simulink model "Final_Tune_of_Bandwidth_PI_Result"  (R2022b)
settings: Solver=FixedStepDiscrete  StartTime=0.0  StopTime=Inf  FixedStep=100e-6  RelTol=1e-3  EnableMultiTasking=on
undefined symbols (not defined in the file): C28x, CPU1, CPU2, CurrentBypassValue, DiscIntNeverNeededParam, Down, GPTRIP1SEL, TZ1, Up
libraries: c2802xlib x20, simulink x16, dspstat3 x10, dspsigops x6, c2837xDlib x5, PID_Lib x5, c280xlib x3, c2000lib x1
(part 3 of 3)

== system Final_Tune_of_Bandwidth_PI_Result/Subsystem5/Subsystem3 ==
  DiffInput : Inport
  Trigger : Inport  Port=2
  Cast1 : DataTypeConversion  OutDataTypeStr=int8  SaturateOnIntegerOverflow=off  RndMeth=Floor
  Mean1 : dspstat3/Mean  run=on  InputProcessing=Columns as channels (frame based)  reset_popup=Rising edge  directionMode=Each column  dimension=1  roiEnable=off  roiType=Rectangles  roiPortion=Entire ROI  roiOutput=Individual statistics for each ROI  roiFlag=off  roundingMode=Floor  overflowMode=off  outputDataTypeStr=Inherit: Same as accumulator  outputMin=[]  outputMax=[]  outputLastDataTypeStr=Inherit: Same as accumulator
  Mean : Outport
  wires:
  Cast1/1 -> Mean1/2
  DiffInput/1 -> Mean1/1
  Mean1/1 -> Mean/1
  Trigger/1 -> Cast1/1

== system Final_Tune_of_Bandwidth_PI_Result/Subsystem5/Subsystem4 ==
  DiffInput : Inport
  Trigger : Inport  Port=2
  Cast1 : DataTypeConversion  OutDataTypeStr=int8  SaturateOnIntegerOverflow=off  RndMeth=Floor
  Mean1 : dspstat3/Mean  run=on  InputProcessing=Columns as channels (frame based)  reset_popup=Rising edge  directionMode=Each column  dimension=1  roiEnable=off  roiType=Rectangles  roiPortion=Entire ROI  roiOutput=Individual statistics for each ROI  roiFlag=off  roundingMode=Floor  overflowMode=off  outputDataTypeStr=Inherit: Same as accumulator  outputMin=[]  outputMax=[]  outputLastDataTypeStr=Inherit: Same as accumulator
  Mean : Outport
  wires:
  Cast1/1 -> Mean1/2
  DiffInput/1 -> Mean1/1
  Mean1/1 -> Mean/1
  Trigger/1 -> Cast1/1

== system Final_Tune_of_Bandwidth_PI_Result/Subsystem5/Subsystem6 ==
  DiffInput : Inport
  Trigger : Inport  Port=2
  Cast1 : DataTypeConversion  OutDataTypeStr=int8  SaturateOnIntegerOverflow=off  RndMeth=Floor
  Mean1 : dspstat3/Mean  run=on  InputProcessing=Columns as channels (frame based)  reset_popup=Rising edge  directionMode=Each column  dimension=1  roiEnable=off  roiType=Rectangles  roiPortion=Entire ROI  roiOutput=Individual statistics for each ROI  roiFlag=off  roundingMode=Floor  overflowMode=off  outputDataTypeStr=Inherit: Same as accumulator  outputMin=[]  outputMax=[]  outputLastDataTypeStr=Inherit: Same as accumulator
  Mean : Outport
  wires:
  Cast1/1 -> Mean1/2
  DiffInput/1 -> Mean1/1
  Mean1/1 -> Mean/1
  Trigger/1 -> Cast1/1

== system Final_Tune_of_Bandwidth_PI_Result/Voltage_Loop/Subsystem5 ==
  MPCC_f32DCLink : Inport
  Cast To Single1 : DataTypeConversion  OutDataTypeStr=single  SaturateOnIntegerOverflow=off  RndMeth=Floor
  LPF : Subsystem
  MPCC_f32DCLinkFiltered : Outport
  wires:
  LPF/1(y_k) -> Cast To Single1/1
  MPCC_f32DCLink/1 -> LPF/1(u_k)
  Cast To Single1/1 -> MPCC_f32DCLinkFiltered/1  "Iau"

== system Final_Tune_of_Bandwidth_PI_Result/Subsystem1/ABCtoDQO/ABCtoDQOCurrent ==
  PI_f32GridCurrentA : Inport
  PI_f32GridCurrentB : Inport  Port=2
  PI_f32GridCurrentC : Inport  Port=3
  PI_f32ElectricalAngle : Inport  Port=4
  ABCtoO : Subsystem
  ABCtoQ : Subsystem
  ABCtoQ1 : Subsystem
  PI_f32DGridCurrent : Outport
  PI_f32QGridCurrent : Outport  Port=2
  PI_f32OGridCurrent : Outport  Port=3
  wires:
  ABCtoQ/1(PI_f32QGridCurrent) -> PI_f32QGridCurrent/1
  [PI_f32GridCurrentC] -> ABCtoQ/3(PI_f32GridCurrentC)
  PI_f32GridCurrentC/1 -> [PI_f32GridCurrentC]
  PI_f32GridCurrentA/1 -> [PI_f32GridCurrentA]
  [PI_f32GridCurrentB] -> ABCtoO/2(PI_f32GridCurrentB)
  [PI_f32GridCurrentA] -> ABCtoO/1(PI_f32GridCurrentA)
  [PI_f32ElectricalAngle] -> ABCtoQ/4(PI_f32ElectricalAngle)
  [PI_f32GridCurrentA] -> ABCtoQ/1(PI_f32GridCurrentA)
  [PI_f32GridCurrentC] -> ABCtoO/3(PI_f32GridCurrentC)
  [PI_f32GridCurrentB] -> ABCtoQ/2(PI_f32GridCurrentB)
  PI_f32ElectricalAngle/1 -> [PI_f32ElectricalAngle]
  PI_f32GridCurrentB/1 -> [PI_f32GridCurrentB]
  ABCtoQ1/1(MPCC_f32QGridVoltage) -> PI_f32DGridCurrent/1
  ABCtoO/1(PI_f32OGridCurrent) -> PI_f32OGridCurrent/1
  [PI_f32GridCurrentA] -> ABCtoQ1/1(MPCC_f32GridVoltageA)
  [PI_f32GridCurrentB] -> ABCtoQ1/2(MPCC_f32GridVoltageB)
  [PI_f32GridCurrentC] -> ABCtoQ1/3(MPCC_f32GridVoltageC)
  [PI_f32ElectricalAngle] -> ABCtoQ1/4(MPCC_f32ElectricalAngle)

== system Final_Tune_of_Bandwidth_PI_Result/Subsystem1/ABCtoDQO/ABCtoDQOVoltage ==
  PI_f32GridCurrentA : Inport
  PI_f32GridCurrentB : Inport  Port=2
  PI_f32GridCurrentC : Inport  Port=3
  PI_f32ElectricalAngle : Inport  Port=4
  ABCtoO : Subsystem
  ABCtoQ : Subsystem
  ABCtoQ1 : Subsystem
  PI_f32DGridCurrent : Outport
  PI_f32QGridCurrent : Outport  Port=2
  PI_f32OGridCurrent : Outport  Port=3
  wires:
  ABCtoQ/1(PI_f32QGridCurrent) -> PI_f32QGridCurrent/1
  [PI_f32GridCurrentC] -> ABCtoQ/3(PI_f32GridCurrentC)
  PI_f32GridCurrentC/1 -> [PI_f32GridCurrentC]
  PI_f32GridCurrentA/1 -> [PI_f32GridCurrentA]
  [PI_f32GridCurrentB] -> ABCtoO/2(PI_f32GridCurrentB)
  [PI_f32GridCurrentA] -> ABCtoO/1(PI_f32GridCurrentA)
  [PI_f32ElectricalAngle] -> ABCtoQ/4(PI_f32ElectricalAngle)
  [PI_f32GridCurrentA] -> ABCtoQ/1(PI_f32GridCurrentA)
  [PI_f32GridCurrentC] -> ABCtoO/3(PI_f32GridCurrentC)
  [PI_f32GridCurrentB] -> ABCtoQ/2(PI_f32GridCurrentB)
  PI_f32ElectricalAngle/1 -> [PI_f32ElectricalAngle]
  PI_f32GridCurrentB/1 -> [PI_f32GridCurrentB]
  ABCtoQ1/1(MPCC_f32QGridVoltage) -> PI_f32DGridCurrent/1
  ABCtoO/1(PI_f32OGridCurrent) -> PI_f32OGridCurrent/1
  [PI_f32GridCurrentA] -> ABCtoQ1/1(MPCC_f32GridVoltageA)
  [PI_f32GridCurrentB] -> ABCtoQ1/2(MPCC_f32GridVoltageB)
  [PI_f32GridCurrentC] -> ABCtoQ1/3(MPCC_f32GridVoltageC)
  [PI_f32ElectricalAngle] -> ABCtoQ1/4(MPCC_f32ElectricalAngle)

== system Final_Tune_of_Bandwidth_PI_Result/Subsystem1/ABCtoDQO/abc_dq ==
  theta : Inport
  a : Inport  Port=2
  b : Inport  Port=3
  c : Inport  Port=4
  Subsystem5 : Subsystem
  Subsystem6 : Subsystem
  Id : Outport
  Iq : Outport  Port=2
  wires:
  c/1 -> Subsystem5/3(In3)
  Subsystem5/2(Out2) -> Subsystem6/2(In2)
  b/1 -> Subsystem5/2(In2)
  theta/1 -> Subsystem6/3(theta)
  Subsystem6/1(Id) -> Id/1
  Subsystem5/1(Out1) -> Subsystem6/1(In1)
  Subsystem6/2(Iq) -> Iq/1
  a/1 -> Subsystem5/1(In1)

== system Final_Tune_of_Bandwidth_PI_Result/Subsystem1/ABCtoDQO/abc_dq1 ==
  theta : Inport
  a : Inport  Port=2
  b : Inport  Port=3
  c : Inport  Port=4
  Subsystem5 : Subsystem
  Subsystem6 : Subsystem
  Id : Outport
  Iq : Outport  Port=2
  wires:
  c/1 -> Subsystem5/3(In3)
  Subsystem5/2(Out2) -> Subsystem6/2(In2)
  b/1 -> Subsystem5/2(In2)
  theta/1 -> Subsystem6/3(theta)
  Subsystem6/1(Id) -> Id/1
  Subsystem5/1(Out1) -> Subsystem6/1(In1)
  Subsystem6/2(Iq) -> Iq/1
  a/1 -> Subsystem5/1(In1)

== system Final_Tune_of_Bandwidth_PI_Result/Subsystem1/Decoupling_Loop/ABCtoDQOVoltage ==
  PI_f32MDVoltageRef : Inport
  PI_f32MQVoltageRef : Inport  Port=2
  PI_f32MOVoltageRef : Inport  Port=3
  PI_f32ElectricalAngle : Inport  Port=4
  DQOtoA : Subsystem
  DQOtoB : Subsystem
  DQOtoC : Subsystem
  PI_f32MAVoltageRef : Outport
  PI_f32MBVoltageRef : Outport  Port=2
  PI_f32MCVoltageRef : Outport  Port=3
  wires:
  [PI_f32MOVoltageRef] -> DQOtoB/3(PI_f32MOVoltageRef)
  [PI_f32MOVoltageRef] -> DQOtoC/3(PI_f32MOVoltageRef)
  [PI_f32ElectricalAngle] -> DQOtoA/4(PI_f32ElectricalAngle)
  [PI_f32ElectricalAngle] -> DQOtoC/4(PI_f32ElectricalAngle)
  [PI_f32ElectricalAngle] -> DQOtoB/4(PI_f32ElectricalAngle)
  [PI_f32MDVoltageRef] -> DQOtoC/1(PI_f32MDVoltageRef)
  [PI_f32MQVoltageRef] -> DQOtoA/2(PI_f32MQVoltageRef)
  [PI_f32MOVoltageRef] -> DQOtoA/3(PI_f32MOVoltageRef)
  [PI_f32MQVoltageRef] -> DQOtoC/2(PI_f32MQVoltageRef)
  [PI_f32MDVoltageRef] -> DQOtoA/1(PI_f32MDVoltageRef)
  [PI_f32MDVoltageRef] -> DQOtoB/1(PI_f32MDVoltageRef)
  [PI_f32MQVoltageRef] -> DQOtoB/2(PI_f32MQVoltageRef)
  DQOtoA/1(PI_f32MAVoltageRef) -> PI_f32MAVoltageRef/1
  DQOtoB/1(PI_f32MBVoltageRef) -> PI_f32MBVoltageRef/1
  DQOtoC/1(PI_f32MCVoltageRef) -> PI_f32MCVoltageRef/1
  PI_f32MDVoltageRef/1 -> [PI_f32MDVoltageRef]
  PI_f32MQVoltageRef/1 -> [PI_f32MQVoltageRef]
  PI_f32MOVoltageRef/1 -> [PI_f32MOVoltageRef]
  PI_f32ElectricalAngle/1 -> [PI_f32ElectricalAngle]

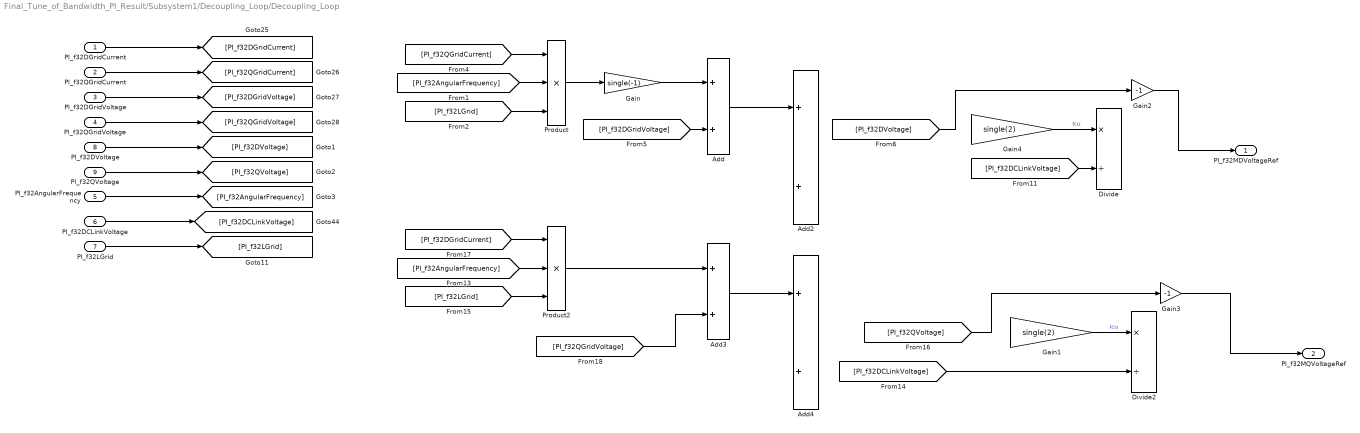
== system Final_Tune_of_Bandwidth_PI_Result/Subsystem1/Decoupling_Loop/Decoupling_Loop ==
  PI_f32DGridCurrent : Inport
  PI_f32QGridCurrent : Inport  Port=2
  PI_f32DGridVoltage : Inport  Port=3
  PI_f32QGridVoltage : Inport  Port=4
  PI_f32AngularFrequency : Inport  Port=5
  PI_f32DCLinkVoltage : Inport  Port=6
  PI_f32LGrid : Inport  Port=7
  PI_f32DVoltage : Inport  Port=8
  PI_f32QVoltage : Inport  Port=9
  Add : Sum
  Add2 : Sum  OutDataTypeStr=single
  Add3 : Sum
  Add4 : Sum  OutDataTypeStr=single
  Divide : Product  Inputs=*/  OutDataTypeStr=single  RndMeth=Zero  SaturateOnIntegerOverflow=on
  Divide2 : Product  Inputs=*/  OutDataTypeStr=single  RndMeth=Zero  SaturateOnIntegerOverflow=on
  Gain : Gain  Gain=single(-1)
  Gain1 : Gain  Gain=single(2)
  Gain2 : Gain  Gain=-1
  Gain3 : Gain  Gain=-1
  Gain4 : Gain  Gain=single(2)
  Product : Product  Inputs=3
  Product2 : Product  Inputs=3
  PI_f32MDVoltageRef : Outport
  PI_f32MQVoltageRef : Outport  Port=2
  wires:
  [PI_f32DCLinkVoltage] -> Divide/2
  PI_f32DGridCurrent/1 -> [PI_f32DGridCurrent]
  PI_f32QVoltage/1 -> [PI_f32QVoltage]
  PI_f32DGridVoltage/1 -> [PI_f32DGridVoltage]
  [PI_f32QGridCurrent] -> Product/1
  Product/1 -> Gain/1
  PI_f32DVoltage/1 -> [PI_f32DVoltage]
  PI_f32LGrid/1 -> [PI_f32LGrid]
  PI_f32DCLinkVoltage/1 -> [PI_f32DCLinkVoltage]
  [PI_f32AngularFrequency] -> Product/2
  PI_f32AngularFrequency/1 -> [PI_f32AngularFrequency]
  PI_f32QGridCurrent/1 -> [PI_f32QGridCurrent]
  [PI_f32LGrid] -> Product/3
  PI_f32QGridVoltage/1 -> [PI_f32QGridVoltage]
  Add/1 -> Add2/1
  ? -> Add2/2
  Product2/1 -> Add3/1
  [PI_f32DCLinkVoltage] -> Divide2/2
  [PI_f32DGridCurrent] -> Product2/1
  [PI_f32LGrid] -> Product2/3
  ? -> Add4/2
  Add3/1 -> Add4/1
  [PI_f32AngularFrequency] -> Product2/2
  Gain/1 -> Add/1
  [PI_f32QGridVoltage] -> Add3/2
  Gain4/1 -> Divide/1  "Icu"
  Gain1/1 -> Divide2/1  "Icu"
  [PI_f32DGridVoltage] -> Add/2
  [PI_f32DVoltage] -> Gain2/1
  [PI_f32QVoltage] -> Gain3/1
  Gain2/1 -> PI_f32MDVoltageRef/1
  Gain3/1 -> PI_f32MQVoltageRef/1

== system Final_Tune_of_Bandwidth_PI_Result/Subsystem1/Decoupling_Loop/dq_abc ==
  theta : Inport
  vd : Inport  Port=2
  vq : Inport  Port=3
  Subsystem6 : Subsystem
  Ia : Outport
  Ib : Outport  Port=2
  Ic : Outport  Port=3
  wires:
  theta/1 -> Subsystem6/3(theta)
  vd/1 -> Subsystem6/1(In1)
  vq/1 -> Subsystem6/2(In2)
  Subsystem6/1(Ia) -> Ia/1
  Subsystem6/2(Ib) -> Ib/1
  Subsystem6/3(Ic) -> Ic/1

== system Final_Tune_of_Bandwidth_PI_Result/Subsystem1/Subsystem1/CodeGeneration ==
  Input : Inport
  Add : Sum  Inputs=+-  OutDataTypeStr=Inherit: Same as first input
  Demux2 : Demux  Outputs=2
  Index Vector : MultiPortSwitch  Inputs=1  SaturateOnIntegerOverflow=off  InputSameDT=off
  SCI Transmit : c280xlib/SCI Transmit  sciModule=A  dataHead=''  dataTail=''  blockingMode=on  outputStatus=off
  While Iterator : WhileIterator  MaxIters=-1  WhileBlockType=do-while  ShowIterationPort=on  OutputDataType=int16
  wires:
  While Iterator/1 -> Add/2, Index Vector/1
  Demux2/1 -> Index Vector/2
  Index Vector/1 -> SCI Transmit/1
  Add/1 -> While Iterator/1
  Demux2/2 -> Add/1
  Input/1 -> Demux2/1

== system Final_Tune_of_Bandwidth_PI_Result/Subsystem1/Subsystem1/Data ==
  Data : Inport
  Data_width : Inport  Port=2
  Action Port : ActionPort  ActionPortLabel=else
  Mux : Mux  Inputs=2
  Start : Constant  Value=hex2dec('0000')  OutDataTypeStr=uint16
  Data_out : Outport  VectorParamsAs1DForOutWhenUnconnected=off
  Iteration : Outport  Port=2  VectorParamsAs1DForOutWhenUnconnected=off
  wires:
  Start/1 -> Mux/2
  Mux/1 -> Data_out/1
  Data/1 -> Mux/1
  Data_width/1 -> Iteration/1

== system Final_Tune_of_Bandwidth_PI_Result/Subsystem1/Subsystem1/Data_Conditioning ==
  In1 : Inport
  Data Type Conversion3 : DataTypeConversion  OutDataTypeStr=uint16  ConvertRealWorld=Stored Integer (SI)  SaturateOnIntegerOverflow=off  RndMeth=Floor
  Out1 : Outport  VectorParamsAs1DForOutWhenUnconnected=off
  wires:
  Data Type Conversion3/1 -> Out1/1
  In1/1 -> Data Type Conversion3/1

== system Final_Tune_of_Bandwidth_PI_Result/Subsystem1/Subsystem1/End ==
  Data : Inport
  Data_width : Inport  Port=2
  Action Port : ActionPort  ActionPortLabel=elseif(u1 == 599)
  Bias : Bias  Bias=1  SaturateOnIntegerOverflow=off
  Mux : Mux  Inputs=2
  Start : Constant  Value=hex2dec('4545')  OutDataTypeStr=uint16
  Data_out : Outport  VectorParamsAs1DForOutWhenUnconnected=off
  Iteration : Outport  Port=2  VectorParamsAs1DForOutWhenUnconnected=off
  wires:
  Mux/1 -> Data_out/1
  Data_width/1 -> Bias/1
  Start/1 -> Mux/2
  Bias/1 -> Iteration/1
  Data/1 -> Mux/1

== system Final_Tune_of_Bandwidth_PI_Result/Subsystem1/Subsystem1/Start ==
  Data : Inport
  Data_width : Inport  Port=2
  Action Port : ActionPort  ActionPortLabel=if(u1 == 0)
  Bias : Bias  Bias=1  SaturateOnIntegerOverflow=off
  End : Constant  Value=hex2dec('5353')  OutDataTypeStr=uint16
  Mux : Mux  Inputs=2
  Data_out : Outport  VectorParamsAs1DForOutWhenUnconnected=off
  Iteration : Outport  Port=2  VectorParamsAs1DForOutWhenUnconnected=off
  wires:
  End/1 -> Mux/1
  Mux/1 -> Data_out/1
  Data_width/1 -> Bias/1
  Bias/1 -> Iteration/1
  Data/1 -> Mux/2

== system Final_Tune_of_Bandwidth_PI_Result/Subsystem3/PLL2/Clarke Transformation1 ==
  va : Inport
  vb : Inport  Port=2
  vc : Inport  Port=3
  Gain1 : Gain  Gain=0.5
  Gain2 : Gain  Gain=0.5
  Gain3 : Gain  Gain=2/3
  Gain4 : Gain  Gain=2/3
  Gain5 : Gain  Gain=sqrt(3)/2
  Sum : Sum  Inputs=+--
  Sum1 : Sum  Inputs=+-
  I_alpha : Outport
  I_beta : Outport  Port=2
  wires:
  Gain1/1 -> Sum/3
  Gain2/1 -> Sum/2
  Gain4/1 -> I_beta/1
  Sum/1 -> Gain3/1
  Gain3/1 -> I_alpha/1
  va/1 -> Sum/1
  Sum1/1 -> Gain5/1
  vc/1 -> Gain1/1, Sum1/2
  Gain5/1 -> Gain4/1
  vb/1 -> Gain2/1, Sum1/1

== system Final_Tune_of_Bandwidth_PI_Result/Subsystem3/PLL2/PhaseMaximumDetector ==
  Va : Inport
  AND1 : Logic  AllPortsSameDT=off  OutDataTypeStr=boolean
  Abs4 : Abs  SaturateOnIntegerOverflow=off
  CycleDetector : Subsystem  TreatAsAtomicUnit=on
  Delay3 : Delay  DelayLength=1
  MinMax Running Resettable3 : simulink/Math Operations/MinMax Running Resettable  Function=max  vinit=0
  NOT1 : Logic  Operator=NOT  AllPortsSameDT=off  OutDataTypeStr=boolean
  Sample and Hold2 : dspsigops/Sample and Hold  trig=Rising edge  initCond=100  latchinput=on
  Zero Crossing4 : dspsigops/Zero Crossing  InputProcessing=Columns as channels (frame based)
  Vamax : Outport
  wires:
  Va/1 -> Abs4/1, Zero Crossing4/1
  Delay3/1 -> NOT1/1
  Sample and Hold2/1 -> Vamax/1
  MinMax Running Resettable3/1 -> Sample and Hold2/1
  Zero Crossing4/1 -> AND1/1, Delay3/1
  AND1/1 -> CycleDetector/Enable
  Abs4/1 -> MinMax Running Resettable3/1
  NOT1/1 -> AND1/2
  CycleDetector/1(Reset) -> [Reset]
  [Reset] -> MinMax Running Resettable3/2
  [Reset] -> Sample and Hold2/Trigger

== system Final_Tune_of_Bandwidth_PI_Result/Subsystem3/PLL2/PhaseMaximumDetector1 ==
  Vb : Inport
  AND1 : Logic  AllPortsSameDT=off  OutDataTypeStr=boolean
  Abs4 : Abs  SaturateOnIntegerOverflow=off
  CycleDetector : Subsystem  TreatAsAtomicUnit=on
  Delay3 : Delay  DelayLength=1
  MinMax Running Resettable3 : simulink/Math Operations/MinMax Running Resettable  Function=max  vinit=0
  NOT1 : Logic  Operator=NOT  AllPortsSameDT=off  OutDataTypeStr=boolean
  Sample and Hold2 : dspsigops/Sample and Hold  trig=Rising edge  initCond=100  latchinput=on
  Zero Crossing4 : dspsigops/Zero Crossing  InputProcessing=Columns as channels (frame based)
  Vbmax : Outport
  wires:
  Vb/1 -> Abs4/1, Zero Crossing4/1
  Delay3/1 -> NOT1/1
  Sample and Hold2/1 -> Vbmax/1
  MinMax Running Resettable3/1 -> Sample and Hold2/1
  Zero Crossing4/1 -> AND1/1, Delay3/1
  AND1/1 -> CycleDetector/Enable
  Abs4/1 -> MinMax Running Resettable3/1
  NOT1/1 -> AND1/2
  CycleDetector/1(Reset) -> [Reset]
  [Reset] -> MinMax Running Resettable3/2
  [Reset] -> Sample and Hold2/Trigger

== system Final_Tune_of_Bandwidth_PI_Result/Subsystem3/PLL2/PhaseMaximumDetector2 ==
  Vc : Inport
  AND1 : Logic  AllPortsSameDT=off  OutDataTypeStr=boolean
  Abs4 : Abs  SaturateOnIntegerOverflow=off
  CycleDetector : Subsystem  TreatAsAtomicUnit=on
  Delay3 : Delay  DelayLength=1
  MinMax Running Resettable3 : simulink/Math Operations/MinMax Running Resettable  Function=max  vinit=0
  NOT1 : Logic  Operator=NOT  AllPortsSameDT=off  OutDataTypeStr=boolean
  Sample and Hold2 : dspsigops/Sample and Hold  trig=Rising edge  initCond=100  latchinput=on
  Zero Crossing4 : dspsigops/Zero Crossing  InputProcessing=Columns as channels (frame based)
  Vcmax : Outport
  wires:
  Vc/1 -> Abs4/1, Zero Crossing4/1
  Delay3/1 -> NOT1/1
  Sample and Hold2/1 -> Vcmax/1
  MinMax Running Resettable3/1 -> Sample and Hold2/1
  Zero Crossing4/1 -> AND1/1, Delay3/1
  AND1/1 -> CycleDetector/Enable
  Abs4/1 -> MinMax Running Resettable3/1
  NOT1/1 -> AND1/2
  CycleDetector/1(Reset) -> [Reset]
  [Reset] -> MinMax Running Resettable3/2
  [Reset] -> Sample and Hold2/Trigger

== system Final_Tune_of_Bandwidth_PI_Result/Subsystem3/PLL_Loop/ABCtoQ ==
  MPCC_f32GridVoltageA : Inport
  MPCC_f32GridVoltageB : Inport  Port=2
  MPCC_f32GridVoltageC : Inport  Port=3
  MPCC_f32ElectricalAngle : Inport  Port=4
  Add : Sum  Inputs=+++
  Add1 : Sum  Inputs=+-
  Add2 : Sum
  Constant : Constant  Value=single(2*pi/3)
  Constant1 : Constant  Value=single(2*pi/3)
  Gain : Gain  Gain=single(-2/3)
  Product : Product
  Product1 : Product
  Product2 : Product
  Sin1 : Trigonometry
  Sin2 : Trigonometry
  Sin3 : Trigonometry
  MPCC_f32QGridVoltage : Outport
  wires:
  [MPCC_f32ElectricalAngle] -> Add2/1
  Sin1/1 -> Product1/2
  MPCC_f32ElectricalAngle/1 -> [MPCC_f32ElectricalAngle]
  Product1/1 -> Add/2
  Constant/1 -> Add1/2
  Product2/1 -> Add/3
  Product/1 -> Add/1
  Add2/1 -> Sin2/1
  Sin2/1 -> Product2/2
  Add1/1 -> Sin1/1
  Constant1/1 -> Add2/2
  Add/1 -> Gain/1
  [MPCC_f32ElectricalAngle] -> Add1/1
  MPCC_f32GridVoltageB/1 -> Product1/1
  [MPCC_f32ElectricalAngle] -> Sin3/1
  MPCC_f32GridVoltageA/1 -> Product/1
  Sin3/1 -> Product/2
  MPCC_f32GridVoltageC/1 -> Product2/1
  Gain/1 -> MPCC_f32QGridVoltage/1

== system Final_Tune_of_Bandwidth_PI_Result/Subsystem3/PLL_Loop1/ABCtoAlphaBeta ==
  In1 : Inport
  In2 : Inport  Port=2
  In3 : Inport  Port=3
  Add : Sum  Inputs=+-
  Add1 : Sum  Inputs=+--
  Gain : Gain  Gain=0.5
  Gain1 : Gain  Gain=sqrt(3)/2
  Gain2 : Gain  Gain=2/3
  Gain3 : Gain  Gain=2/3
  Gain4 : Gain  Gain=0.5
  Out1 : Outport
  Vαβ : Outport  Port=2
  wires:
  In1/1 -> Add1/1
  Gain4/1 -> Add1/3
  Gain/1 -> Add1/2
  In2/1 -> Add/1, Gain/1
  In3/1 -> Add/2, Gain4/1
  Add/1 -> Gain1/1
  Add1/1 -> Gain2/1
  Gain2/1 -> Out1/1
  Gain1/1 -> Gain3/1
  Gain3/1 -> Vαβ/1

== system Final_Tune_of_Bandwidth_PI_Result/Subsystem3/PLL_Loop1/Discrete integrator 2π wrapping1 ==
  ω : Inport
  Compare To Constant : simulink/Logic and Bit Operations/Compare To Constant  relop=<  const=0  OutDataTypeStr=boolean
  Compare To Constant1 : simulink/Logic and Bit Operations/Compare To Constant  relop=>=  const=2*pi  OutDataTypeStr=boolean
  Discrete-Time Integrator : DiscreteIntegrator  ExternalReset=sampled level  InitialConditionSource=external  SampleTime=-1  ShowStatePort=on  ICPrevOutput=DiscIntNeverNeededParam  ICPrevScaledInput=DiscIntNeverNeededParam
  Gain : Gain  Gain=1/(2*pi)
      settings: AttributesFormatString=%<Gain>
  Gain1 : Gain  Gain=2*pi
  IC : InitialCondition  Value=0
  Logical Operator : Logic  Operator=OR  AllPortsSameDT=off  OutDataTypeStr=boolean
  Rounding Function : Rounding
  Sum1 : Sum  Inputs=|+-
  θ : Outport
  wires:
  Gain1/1 -> Sum1/2
  Gain/1 -> Rounding Function/1
  IC/1 -> Discrete-Time Integrator/3
  Compare To Constant1/1 -> Logical Operator/2
  Discrete-Time Integrator/State -> Compare To Constant1/1, Sum1/1, Gain/1, Compare To Constant/1
  Compare To Constant/1 -> Logical Operator/1
  Logical Operator/1 -> Discrete-Time Integrator/2
  Sum1/1 -> IC/1
  Rounding Function/1 -> Gain1/1
  ω/1 -> Discrete-Time Integrator/1
  Discrete-Time Integrator/1 -> θ/1

== system Final_Tune_of_Bandwidth_PI_Result/Subsystem3/PLL_Loop1/SOGI 1st ==
  w : Inport
  Vαβ : Inport  Port=2
  Gain : Gain  Gain=sqrt(2)  OutDataTypeStr=single
  Gain1 : Gain  Gain=0  OutDataTypeStr=single
  Integrator : Subsystem
  Integrator1 : Subsystem
  Integrator2 : Subsystem
  Multiply : Product
  Multiply1 : Product
  Multiply2 : Product
  Saturation : Saturate  UpperLimit=5  LowerLimit=-5
  Sum : Sum  Inputs=-+|
  Sum1 : Sum  Inputs=|+-
  Sum2 : Sum  Inputs=++|
  v : Outport
  qv : Outport  Port=2  OutDataTypeStr=single
  wires:
  w/1 -> Multiply2/2, Multiply/2, Multiply1/1
  Sum/1 -> Saturation/1, Gain/1
  Gain/1 -> Sum1/1
  Vαβ/1 -> Sum/2
  Sum1/1 -> Multiply/1
  Multiply/1 -> Integrator/1(In)
  Multiply2/1 -> Integrator2/1(In)
  Gain1/1 -> Multiply2/1
  Saturation/1 -> Gain1/1
  Integrator/1(Out) -> Sum2/2, v/1, Integrator1/1(In)
  Integrator1/1(Out) -> Multiply1/2
  Multiply1/1 -> Sum1/2, qv/1
  Integrator2/1(Out) -> Sum2/1
  Sum2/1 -> Sum/1

== system Final_Tune_of_Bandwidth_PI_Result/Subsystem3/PLL_Loop1/SOGI 1st2 ==
  w : Inport
  Vαβ : Inport  Port=2
  Cast To Single : DataTypeConversion  OutDataTypeStr=single  SaturateOnIntegerOverflow=off  RndMeth=Floor
  Delay One Step : Delay  DelayLength=1  InitialCondition=0.5
  Delay One Step1 : Delay  DelayLength=1  InitialCondition=-0.5
  Gain : Gain  Gain=sqrt(2)  OutDataTypeStr=single
  Gain1 : Gain  Gain=100e-6  OutDataTypeStr=single
  Multiply1 : Product
  Product : Product
  Sum : Sum  Inputs=-+|
  Sum1 : Sum  Inputs=|+-
  Sum2 : Sum  Inputs=++|
  Sum3 : Sum  Inputs=++|
  v : Outport
  qv : Outport  Port=2  OutDataTypeStr=single
  wires:
  Sum/1 -> Gain/1
  Gain/1 -> Sum1/1
  Vαβ/1 -> Sum/2
  w/1 -> Gain1/1
  Sum1/1 -> Product/2
  Gain1/1 -> [WTs], Product/1
  Product/1 -> Sum2/2
  Sum2/1 -> Cast To Single/1, Delay One Step/1, v/1
  Delay One Step/1 -> Sum2/1, Sum/1
  [WTs] -> Multiply1/2
  Multiply1/1 -> Sum3/2
  Delay One Step1/1 -> Sum3/1, Sum1/2
  Sum3/1 -> Delay One Step1/1, qv/1
  Cast To Single/1 -> Multiply1/1

== system Final_Tune_of_Bandwidth_PI_Result/Subsystem3/PLL_Loop1/SOGI 1st3 ==
  w : Inport
  Vαβ : Inport  Port=2
  Gain : Gain  Gain=sqrt(2)  OutDataTypeStr=single
  Gain1 : Gain  Gain=0  OutDataTypeStr=single
  Integrator : Subsystem
  Integrator1 : Subsystem
  Integrator2 : Subsystem
  Multiply : Product
  Multiply1 : Product
  Multiply2 : Product
  Saturation : Saturate  UpperLimit=5  LowerLimit=-5
  Sum : Sum  Inputs=-+|
  Sum1 : Sum  Inputs=|+-
  Sum2 : Sum  Inputs=++|
  v : Outport
  qv : Outport  Port=2  OutDataTypeStr=single
  wires:
  w/1 -> Multiply2/2, Multiply/2, Multiply1/1
  Sum/1 -> Saturation/1, Gain/1
  Gain/1 -> Sum1/1
  Vαβ/1 -> Sum/2
  Sum1/1 -> Multiply/1
  Multiply/1 -> Integrator/1(In)
  Multiply2/1 -> Integrator2/1(In)
  Gain1/1 -> Multiply2/1
  Saturation/1 -> Gain1/1
  Integrator/1(Out) -> Sum2/2, v/1, Integrator1/1(In)
  Integrator1/1(Out) -> Multiply1/2
  Multiply1/1 -> Sum1/2, qv/1
  Integrator2/1(Out) -> Sum2/1
  Sum2/1 -> Sum/1

== system Final_Tune_of_Bandwidth_PI_Result/Subsystem3/PLL_Loop1/SOGI 1st4 ==
  w : Inport
  Vαβ : Inport  Port=2
  Cast To Single : DataTypeConversion  OutDataTypeStr=single  SaturateOnIntegerOverflow=off  RndMeth=Floor
  Delay One Step : Delay  DelayLength=1  InitialCondition=0.5
  Delay One Step1 : Delay  DelayLength=1  InitialCondition=-0.5
  Gain : Gain  Gain=sqrt(2)  OutDataTypeStr=single
  Gain1 : Gain  Gain=100e-6  OutDataTypeStr=single
  Multiply1 : Product
  Product : Product
  Sum : Sum  Inputs=-+|
  Sum1 : Sum  Inputs=|+-
  Sum2 : Sum  Inputs=++|
  Sum3 : Sum  Inputs=++|
  v : Outport
  qv : Outport  Port=2  OutDataTypeStr=single
  wires:
  Sum/1 -> Gain/1
  Gain/1 -> Sum1/1
  Vαβ/1 -> Sum/2
  w/1 -> Gain1/1
  Sum1/1 -> Product/2
  Gain1/1 -> [WTs], Product/1
  Product/1 -> Sum2/2
  Sum2/1 -> Cast To Single/1, Delay One Step/1, v/1
  Delay One Step/1 -> Sum2/1, Sum/1
  [WTs] -> Multiply1/2
  Multiply1/1 -> Sum3/2
  Delay One Step1/1 -> Sum3/1, Sum1/2
  Sum3/1 -> Delay One Step1/1, qv/1
  Cast To Single/1 -> Multiply1/1

== system Final_Tune_of_Bandwidth_PI_Result/Subsystem3/PLL_Loop1/Subsystem6 ==
  In1 : Inport
  In2 : Inport  Port=2
  theta : Inport  Port=3
  Add : Sum
  Add1 : Sum  Inputs=-+
  Cos : Trigonometry  Operator=cos
  Cos1 : Trigonometry
  From : From
  From4 : From
  Goto : Goto
  Product{,1..3} (4 alike) : Product
  Id : Outport
  Iq : Outport  Port=2
  wires:
  theta/1 -> Cos1/1, Cos/1
  In1/1 -> Goto/1
  In2/1 -> [b]
  From/1 -> Product/1
  Cos/1 -> [cosine]
  Cos1/1 -> [sinee]
  [cosine] -> Product/2
  [b] -> Product1/1
  [sinee] -> Product1/2
  Product/1 -> Add/1
  Product1/1 -> Add/2
  Add/1 -> Id/1
  [sinee] -> Product2/2
  [b] -> Product3/1
  Product3/1 -> Add1/2
  From4/1 -> Product2/1
  Product2/1 -> Add1/1
  [cosine] -> Product3/2
  Add1/1 -> Iq/1

== system Final_Tune_of_Bandwidth_PI_Result/Voltage_Loop/Subsystem5/LPF ==
  u_k : Inport
  Add : Sum  Inputs=+-
  Add1 : Sum
  Delay : Delay  DelayLength=1
  Gain : Gain  Gain=single(1000/11000)
  y_k : Outport
  wires:
  Delay/1 -> Add/2, Add1/2
  Add/1 -> Gain/1
  Gain/1 -> Add1/1
  Add1/1 -> y_k/1, Delay/1
  u_k/1 -> Add/1

== system Final_Tune_of_Bandwidth_PI_Result/Subsystem1/ABCtoDQO/ABCtoDQOCurrent/ABCtoO ==
  PI_f32GridCurrentA : Inport
  PI_f32GridCurrentB : Inport  Port=2
  PI_f32GridCurrentC : Inport  Port=3
  Add : Sum  Inputs=+++
  Constant1 : Constant  Value=single(1/2)
  Constant2 : Constant  Value=single(1/2)
  Constant3 : Constant  Value=single(1/2)
  Gain : Gain  Gain=single(2/3)
  Product : Product
  Product1 : Product
  Product2 : Product
  PI_f32OGridCurrent : Outport
  wires:
  Product1/1 -> Add/2
  Product2/1 -> Add/3
  Product/1 -> Add/1
  Add/1 -> Gain/1
  PI_f32GridCurrentB/1 -> Product1/1
  PI_f32GridCurrentA/1 -> Product/1
  Constant2/1 -> Product/2
  PI_f32GridCurrentC/1 -> Product2/1
  Constant3/1 -> Product1/2
  Constant1/1 -> Product2/2
  Gain/1 -> PI_f32OGridCurrent/1

== system Final_Tune_of_Bandwidth_PI_Result/Subsystem1/ABCtoDQO/ABCtoDQOCurrent/ABCtoQ ==
  PI_f32GridCurrentA : Inport
  PI_f32GridCurrentB : Inport  Port=2
  PI_f32GridCurrentC : Inport  Port=3
  PI_f32ElectricalAngle : Inport  Port=4
  Add : Sum  Inputs=+++
  Add1 : Sum  Inputs=+-
  Add2 : Sum
  Constant : Constant  Value=single(2*pi/3)
  Constant1 : Constant  Value=single(2*pi/3)
  Gain : Gain  Gain=single(2/3)
  Product : Product
  Product1 : Product
  Product2 : Product
  Sin1 : Trigonometry  Operator=cos
  Sin2 : Trigonometry  Operator=cos
  Sin3 : Trigonometry  Operator=cos
  PI_f32QGridCurrent : Outport
  wires:
  [PI_f32ElectricalAngle] -> Add2/1
  Sin1/1 -> Product1/2
  PI_f32ElectricalAngle/1 -> [PI_f32ElectricalAngle]
  Product1/1 -> Add/2
  Constant/1 -> Add1/2
  Product2/1 -> Add/3
  Product/1 -> Add/1
  Add2/1 -> Sin2/1
  Sin2/1 -> Product2/2
  Add1/1 -> Sin1/1
  Constant1/1 -> Add2/2
  Add/1 -> Gain/1
  [PI_f32ElectricalAngle] -> Add1/1
  PI_f32GridCurrentB/1 -> Product1/1
  [PI_f32ElectricalAngle] -> Sin3/1
  PI_f32GridCurrentA/1 -> Product/1
  Sin3/1 -> Product/2
  PI_f32GridCurrentC/1 -> Product2/1
  Gain/1 -> PI_f32QGridCurrent/1

== system Final_Tune_of_Bandwidth_PI_Result/Subsystem1/ABCtoDQO/ABCtoDQOCurrent/ABCtoQ1 ==
  MPCC_f32GridVoltageA : Inport
  MPCC_f32GridVoltageB : Inport  Port=2
  MPCC_f32GridVoltageC : Inport  Port=3
  MPCC_f32ElectricalAngle : Inport  Port=4
  Add : Sum  Inputs=+++
  Add1 : Sum  Inputs=+-
  Add2 : Sum
  Constant : Constant  Value=single(2*pi/3)
  Constant1 : Constant  Value=single(2*pi/3)
  Gain : Gain  Gain=single(2/3)
  Product : Product
  Product1 : Product
  Product2 : Product
  Sin1 : Trigonometry
  Sin2 : Trigonometry
  Sin3 : Trigonometry
  MPCC_f32QGridVoltage : Outport
  wires:
  [MPCC_f32ElectricalAngle] -> Add2/1
  Sin1/1 -> Product1/2
  MPCC_f32ElectricalAngle/1 -> [MPCC_f32ElectricalAngle]
  Product1/1 -> Add/2
  Constant/1 -> Add1/2
  Product2/1 -> Add/3
  Product/1 -> Add/1
  Add2/1 -> Sin2/1
  Sin2/1 -> Product2/2
  Add1/1 -> Sin1/1
  Constant1/1 -> Add2/2
  Add/1 -> Gain/1
  [MPCC_f32ElectricalAngle] -> Add1/1
  MPCC_f32GridVoltageB/1 -> Product1/1
  [MPCC_f32ElectricalAngle] -> Sin3/1
  MPCC_f32GridVoltageA/1 -> Product/1
  Sin3/1 -> Product/2
  MPCC_f32GridVoltageC/1 -> Product2/1
  Gain/1 -> MPCC_f32QGridVoltage/1

== system Final_Tune_of_Bandwidth_PI_Result/Subsystem1/ABCtoDQO/ABCtoDQOVoltage/ABCtoO ==
  PI_f32GridCurrentA : Inport
  PI_f32GridCurrentB : Inport  Port=2
  PI_f32GridCurrentC : Inport  Port=3
  Add : Sum  Inputs=+++
  Constant1 : Constant  Value=single(1/2)
  Constant2 : Constant  Value=single(1/2)
  Constant3 : Constant  Value=single(1/2)
  Gain : Gain  Gain=single(2/3)
  Product : Product
  Product1 : Product
  Product2 : Product
  PI_f32OGridCurrent : Outport
  wires:
  Product1/1 -> Add/2
  Product2/1 -> Add/3
  Product/1 -> Add/1
  Add/1 -> Gain/1
  PI_f32GridCurrentB/1 -> Product1/1
  PI_f32GridCurrentA/1 -> Product/1
  Constant2/1 -> Product/2
  PI_f32GridCurrentC/1 -> Product2/1
  Constant3/1 -> Product1/2
  Constant1/1 -> Product2/2
  Gain/1 -> PI_f32OGridCurrent/1

== system Final_Tune_of_Bandwidth_PI_Result/Subsystem1/ABCtoDQO/ABCtoDQOVoltage/ABCtoQ ==
  PI_f32GridCurrentA : Inport
  PI_f32GridCurrentB : Inport  Port=2
  PI_f32GridCurrentC : Inport  Port=3
  PI_f32ElectricalAngle : Inport  Port=4
  Add : Sum  Inputs=+++
  Add1 : Sum  Inputs=+-
  Add2 : Sum
  Constant : Constant  Value=single(2*pi/3)
  Constant1 : Constant  Value=single(2*pi/3)
  Gain : Gain  Gain=single(-2/3)
  Product : Product
  Product1 : Product
  Product2 : Product
  Sin1 : Trigonometry
  Sin2 : Trigonometry
  Sin3 : Trigonometry
  PI_f32QGridCurrent : Outport
  wires:
  [PI_f32ElectricalAngle] -> Add2/1
  Sin1/1 -> Product1/2
  PI_f32ElectricalAngle/1 -> [PI_f32ElectricalAngle]
  Product1/1 -> Add/2
  Constant/1 -> Add1/2
  Product2/1 -> Add/3
  Product/1 -> Add/1
  Add2/1 -> Sin2/1
  Sin2/1 -> Product2/2
  Add1/1 -> Sin1/1
  Constant1/1 -> Add2/2
  Add/1 -> Gain/1
  [PI_f32ElectricalAngle] -> Add1/1
  PI_f32GridCurrentB/1 -> Product1/1
  [PI_f32ElectricalAngle] -> Sin3/1
  PI_f32GridCurrentA/1 -> Product/1
  Sin3/1 -> Product/2
  PI_f32GridCurrentC/1 -> Product2/1
  Gain/1 -> PI_f32QGridCurrent/1

== system Final_Tune_of_Bandwidth_PI_Result/Subsystem1/ABCtoDQO/ABCtoDQOVoltage/ABCtoQ1 ==
  MPCC_f32GridVoltageA : Inport
  MPCC_f32GridVoltageB : Inport  Port=2
  MPCC_f32GridVoltageC : Inport  Port=3
  MPCC_f32ElectricalAngle : Inport  Port=4
  Add : Sum  Inputs=+++
  Add1 : Sum  Inputs=+-
  Add2 : Sum
  Constant : Constant  Value=single(2*pi/3)
  Constant1 : Constant  Value=single(2*pi/3)
  Gain : Gain  Gain=single(2/3)
  Product : Product
  Product1 : Product
  Product2 : Product
  Sin1 : Trigonometry  Operator=cos
  Sin2 : Trigonometry  Operator=cos
  Sin3 : Trigonometry  Operator=cos
  MPCC_f32QGridVoltage : Outport
  wires:
  [MPCC_f32ElectricalAngle] -> Add2/1
  Sin1/1 -> Product1/2
  MPCC_f32ElectricalAngle/1 -> [MPCC_f32ElectricalAngle]
  Product1/1 -> Add/2
  Constant/1 -> Add1/2
  Product2/1 -> Add/3
  Product/1 -> Add/1
  Add2/1 -> Sin2/1
  Sin2/1 -> Product2/2
  Add1/1 -> Sin1/1
  Constant1/1 -> Add2/2
  Add/1 -> Gain/1
  [MPCC_f32ElectricalAngle] -> Add1/1
  MPCC_f32GridVoltageB/1 -> Product1/1
  [MPCC_f32ElectricalAngle] -> Sin3/1
  MPCC_f32GridVoltageA/1 -> Product/1
  Sin3/1 -> Product/2
  MPCC_f32GridVoltageC/1 -> Product2/1
  Gain/1 -> MPCC_f32QGridVoltage/1

== system Final_Tune_of_Bandwidth_PI_Result/Subsystem1/ABCtoDQO/abc_dq/Subsystem5 ==
  In1 : Inport
  In2 : Inport  Port=2
  In3 : Inport  Port=3
  Add : Sum  Inputs=+-
  Add1 : Sum  Inputs=+--
  Gain : Gain  Gain=0.5
  Gain1 : Gain  Gain=sqrt(3)/2
  Gain2 : Gain  Gain=2/3
  Gain3 : Gain  Gain=2/3
  Gain4 : Gain  Gain=0.5
  Out1 : Outport
  Out2 : Outport  Port=2
  wires:
  In1/1 -> Add1/1
  Gain4/1 -> Add1/3
  Gain/1 -> Add1/2
  In2/1 -> Add/1, Gain/1
  In3/1 -> Add/2, Gain4/1
  Add/1 -> Gain1/1
  Add1/1 -> Gain2/1
  Gain2/1 -> Out1/1
  Gain1/1 -> Gain3/1
  Gain3/1 -> Out2/1

== system Final_Tune_of_Bandwidth_PI_Result/Subsystem1/ABCtoDQO/abc_dq/Subsystem6 ==
  In1 : Inport
  In2 : Inport  Port=2
  theta : Inport  Port=3
  Add : Sum
  Add1 : Sum  Inputs=-+
  Cos : Trigonometry  Operator=cos
  Cos1 : Trigonometry
  From : From
  From4 : From
  Goto : Goto
  Product{,1..3} (4 alike) : Product
  Id : Outport
  Iq : Outport  Port=2
  wires:
  theta/1 -> Cos1/1, Cos/1
  In1/1 -> Goto/1
  In2/1 -> [b]
  From/1 -> Product/1
  Cos/1 -> [cosine]
  Cos1/1 -> [sinee]
  [cosine] -> Product/2
  [b] -> Product1/1
  [sinee] -> Product1/2
  Product/1 -> Add/1
  Product1/1 -> Add/2
  Add/1 -> Id/1
  [sinee] -> Product2/2
  [b] -> Product3/1
  Product3/1 -> Add1/2
  From4/1 -> Product2/1
  Product2/1 -> Add1/1
  [cosine] -> Product3/2
  Add1/1 -> Iq/1

== system Final_Tune_of_Bandwidth_PI_Result/Subsystem1/ABCtoDQO/abc_dq1/Subsystem5 ==
  In1 : Inport
  In2 : Inport  Port=2
  In3 : Inport  Port=3
  Add : Sum  Inputs=+-
  Add1 : Sum  Inputs=+--
  Gain : Gain  Gain=0.5
  Gain1 : Gain  Gain=sqrt(3)/2
  Gain2 : Gain  Gain=2/3
  Gain3 : Gain  Gain=2/3
  Gain4 : Gain  Gain=0.5
  Out1 : Outport
  Out2 : Outport  Port=2
  wires:
  In1/1 -> Add1/1
  Gain4/1 -> Add1/3
  Gain/1 -> Add1/2
  In2/1 -> Add/1, Gain/1
  In3/1 -> Add/2, Gain4/1
  Add/1 -> Gain1/1
  Add1/1 -> Gain2/1
  Gain2/1 -> Out1/1
  Gain1/1 -> Gain3/1
  Gain3/1 -> Out2/1

== system Final_Tune_of_Bandwidth_PI_Result/Subsystem1/ABCtoDQO/abc_dq1/Subsystem6 ==
  In1 : Inport
  In2 : Inport  Port=2
  theta : Inport  Port=3
  Add : Sum
  Add1 : Sum  Inputs=-+
  Cos : Trigonometry  Operator=cos
  Cos1 : Trigonometry
  From : From
  From4 : From
  Goto : Goto
  Product{,1..3} (4 alike) : Product
  Id : Outport
  Iq : Outport  Port=2
  wires:
  theta/1 -> Cos1/1, Cos/1
  In1/1 -> Goto/1
  In2/1 -> [b]
  From/1 -> Product/1
  Cos/1 -> [cosine]
  Cos1/1 -> [sinee]
  [cosine] -> Product/2
  [b] -> Product1/1
  [sinee] -> Product1/2
  Product/1 -> Add/1
  Product1/1 -> Add/2
  Add/1 -> Id/1
  [sinee] -> Product2/2
  [b] -> Product3/1
  Product3/1 -> Add1/2
  From4/1 -> Product2/1
  Product2/1 -> Add1/1
  [cosine] -> Product3/2
  Add1/1 -> Iq/1

== system Final_Tune_of_Bandwidth_PI_Result/Subsystem1/Decoupling_Loop/ABCtoDQOVoltage/DQOtoA ==
  PI_f32MDVoltageRef : Inport
  PI_f32MQVoltageRef : Inport  Port=2
  PI_f32MOVoltageRef : Inport  Port=3
  PI_f32ElectricalAngle : Inport  Port=4
  Add : Sum  Inputs=+++  OutDataTypeStr=single
  Constant1 : Constant  Value=single(1)
  Gain : Gain  Gain=single(1)
  Gain1 : Gain  Gain=single(1)
  Product : Product
  Product1 : Product
  Product2 : Product
  Saturation1 : Saturate  UpperLimit=1  LowerLimit=-1  ZeroCross=off
  Sin1 : Trigonometry  Operator=cos
  Sin3 : Trigonometry
  PI_f32MAVoltageRef : Outport
  wires:
  Sin1/1 -> Product1/2
  PI_f32ElectricalAngle/1 -> [PI_f32ElectricalAngle]
  Product1/1 -> Gain1/1
  Product2/1 -> Add/3
  Product/1 -> Add/1
  Constant1/1 -> Product2/2
  [PI_f32ElectricalAngle] -> Sin1/1
  Add/1 -> Gain/1
  PI_f32MQVoltageRef/1 -> Product1/1
  [PI_f32ElectricalAngle] -> Sin3/1
  PI_f32MDVoltageRef/1 -> Product/1
  Sin3/1 -> Product/2
  PI_f32MOVoltageRef/1 -> Product2/1
  Gain/1 -> Saturation1/1
  Saturation1/1 -> PI_f32MAVoltageRef/1
  Gain1/1 -> Add/2

== system Final_Tune_of_Bandwidth_PI_Result/Subsystem1/Decoupling_Loop/ABCtoDQOVoltage/DQOtoB ==
  PI_f32MDVoltageRef : Inport
  PI_f32MQVoltageRef : Inport  Port=2
  PI_f32MOVoltageRef : Inport  Port=3
  PI_f32ElectricalAngle : Inport  Port=4
  Add : Sum  Inputs=+++  OutDataTypeStr=single
  Add1 : Sum  Inputs=+-
  Add3 : Sum  Inputs=+-
  Constant : Constant  Value=single(2*pi/3)
  Constant1 : Constant  Value=single(1)
  Constant2 : Constant  Value=single(2*pi/3)
  Gain : Gain  Gain=single(1)
  Gain1 : Gain  Gain=single(1)
  Product : Product
  Product1 : Product
  Product2 : Product
  Saturation1 : Saturate  UpperLimit=1  LowerLimit=-1  ZeroCross=off
  Sin1 : Trigonometry  Operator=cos
  Sin3 : Trigonometry
  PI_f32MBVoltageRef : Outport
  wires:
  Sin1/1 -> Product1/2
  PI_f32ElectricalAngle/1 -> [PI_f32ElectricalAngle]
  Product1/1 -> Gain1/1
  Constant/1 -> Add1/2
  Product2/1 -> Add/3
  Product/1 -> Add/1
  Constant1/1 -> Product2/2
  Add1/1 -> Sin1/1
  Add/1 -> Gain/1
  [PI_f32ElectricalAngle] -> Add1/1
  PI_f32MQVoltageRef/1 -> Product1/1
  PI_f32MDVoltageRef/1 -> Product/1
  Sin3/1 -> Product/2
  PI_f32MOVoltageRef/1 -> Product2/1
  Gain/1 -> Saturation1/1
  Constant2/1 -> Add3/2
  [PI_f32ElectricalAngle] -> Add3/1
  Add3/1 -> Sin3/1
  Saturation1/1 -> PI_f32MBVoltageRef/1
  Gain1/1 -> Add/2

== system Final_Tune_of_Bandwidth_PI_Result/Subsystem1/Decoupling_Loop/ABCtoDQOVoltage/DQOtoC ==
  PI_f32MDVoltageRef : Inport
  PI_f32MQVoltageRef : Inport  Port=2
  PI_f32MOVoltageRef : Inport  Port=3
  PI_f32ElectricalAngle : Inport  Port=4
  Add : Sum  Inputs=+++  OutDataTypeStr=single
  Add1 : Sum
  Add3 : Sum
  Constant : Constant  Value=single(2*pi/3)
  Constant1 : Constant  Value=single(1)
  Constant2 : Constant  Value=single(2*pi/3)
  Gain : Gain  Gain=single(1)
  Gain1 : Gain  Gain=single(1)
  Product : Product  OutDataTypeStr=Inherit: Inherit via back propagation
  Product1 : Product  OutDataTypeStr=Inherit: Inherit via back propagation
  Product2 : Product  OutDataTypeStr=Inherit: Inherit via back propagation
  Saturation1 : Saturate  UpperLimit=1  LowerLimit=-1  ZeroCross=off
  Sin1 : Trigonometry  Operator=cos
  Sin3 : Trigonometry
  PI_f32MCVoltageRef : Outport
  wires:
  Sin1/1 -> Product1/2
  PI_f32ElectricalAngle/1 -> [PI_f32ElectricalAngle]
  Product1/1 -> Gain1/1
  Constant/1 -> Add1/2
  Product2/1 -> Add/3
  Product/1 -> Add/1
  Constant1/1 -> Product2/2
  Add1/1 -> Sin1/1
  Add/1 -> Gain/1
  [PI_f32ElectricalAngle] -> Add1/1
  PI_f32MQVoltageRef/1 -> Product1/1
  PI_f32MDVoltageRef/1 -> Product/1
  Sin3/1 -> Product/2
  PI_f32MOVoltageRef/1 -> Product2/1
  Gain/1 -> Saturation1/1
  Constant2/1 -> Add3/2
  [PI_f32ElectricalAngle] -> Add3/1
  Add3/1 -> Sin3/1
  Saturation1/1 -> PI_f32MCVoltageRef/1
  Gain1/1 -> Add/2

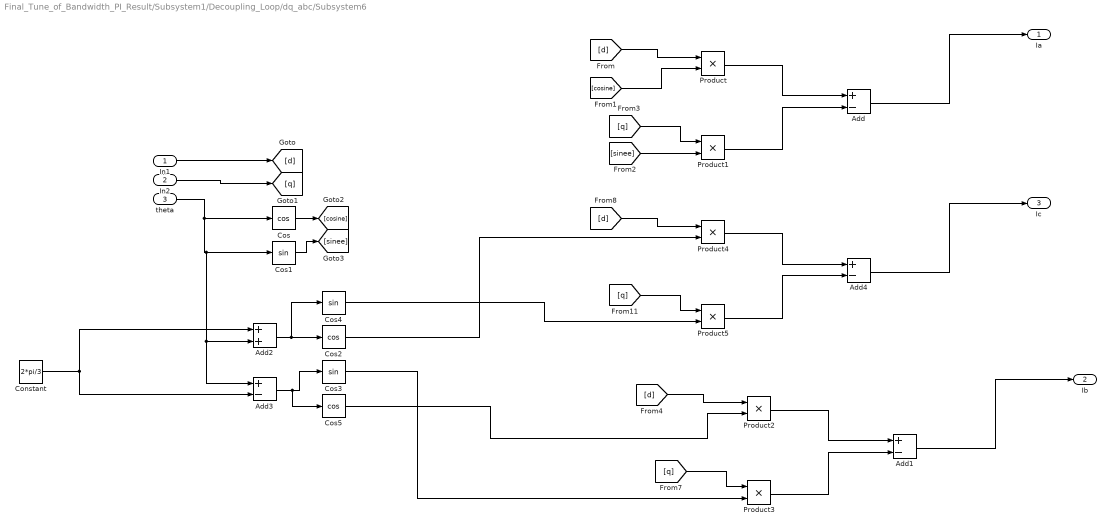
== system Final_Tune_of_Bandwidth_PI_Result/Subsystem1/Decoupling_Loop/dq_abc/Subsystem6 ==
  In1 : Inport
  In2 : Inport  Port=2
  theta : Inport  Port=3
  Add{,1,3..4} (4 alike) : Sum  Inputs=+-
  Add2 : Sum
  Constant : Constant  Value=2*pi/3
  Cos : Trigonometry  Operator=cos
  Cos1 : Trigonometry
  Cos2 : Trigonometry  Operator=cos
  Cos3 : Trigonometry
  Cos4 : Trigonometry
  Cos5 : Trigonometry  Operator=cos
  Product{,1..5} (6 alike) : Product
  Ia : Outport
  Ib : Outport  Port=2
  Ic : Outport  Port=3
  wires:
  theta/1 -> Add2/2, Add3/1, Cos1/1, Cos/1
  In1/1 -> [d]
  In2/1 -> [q]
  [d] -> Product/1
  Cos/1 -> [cosine]
  Cos1/1 -> [sinee]
  [cosine] -> Product/2
  [q] -> Product1/1
  [sinee] -> Product1/2
  Product/1 -> Add/1
  Product1/1 -> Add/2
  Add/1 -> Ia/1
  Constant/1 -> Add3/2, Add2/1
  Add2/1 -> Cos4/1, Cos2/1
  Add3/1 -> Cos5/1, Cos3/1
  Add1/1 -> Ib/1
  [d] -> Product2/1
  Cos3/1 -> Product3/2
  Product3/1 -> Add1/2
  [q] -> Product3/1
  Product2/1 -> Add1/1
  Cos5/1 -> Product2/2
  [q] -> Product5/1
  [d] -> Product4/1
  Product4/1 -> Add4/1
  Add4/1 -> Ic/1
  Cos4/1 -> Product5/2
  Product5/1 -> Add4/2
  Cos2/1 -> Product4/2

== system Final_Tune_of_Bandwidth_PI_Result/Subsystem3/PLL2/PhaseMaximumDetector/CycleDetector ==
  Enable : EnablePort
  Add1 : Sum
  Constant1 : Constant  Value=single(0)
  Constant2 : Constant  Value=single(1)
  Constant6 : Constant  Value=single(2)
  Delay : Delay  DelayLength=1
  Delay One Step : Delay  DelayLength=1  ExternalReset=Rising
      settings: InputPortMap=u0,r5
  GreaterThanOrEqual : RelationalOperator  Operator===  OutDataTypeStr=boolean  RndMeth=Simplest  InputSameDT=off
  Switch1 : Switch  Criteria=u2 > Threshold  SaturateOnIntegerOverflow=off  InputSameDT=off
  Reset : Outport
  wires:
  Delay/1 -> Delay One Step/2
  Constant6/1 -> GreaterThanOrEqual/1
  Delay One Step/1 -> Add1/2, GreaterThanOrEqual/2
  GreaterThanOrEqual/1 -> Reset/1, Delay/1, Switch1/2
  Constant1/1 -> Switch1/1
  Add1/1 -> Delay One Step/1
  Constant2/1 -> Switch1/3
  Switch1/1 -> Add1/1

== system Final_Tune_of_Bandwidth_PI_Result/Subsystem3/PLL2/PhaseMaximumDetector1/CycleDetector ==
  Enable : EnablePort
  Add1 : Sum
  Constant1 : Constant  Value=single(0)
  Constant2 : Constant  Value=single(1)
  Constant6 : Constant  Value=single(2)
  Delay : Delay  DelayLength=1
  Delay One Step : Delay  DelayLength=1  ExternalReset=Rising
      settings: InputPortMap=u0,r5
  GreaterThanOrEqual : RelationalOperator  Operator===  OutDataTypeStr=boolean  RndMeth=Simplest  InputSameDT=off
  Switch1 : Switch  Criteria=u2 > Threshold  SaturateOnIntegerOverflow=off  InputSameDT=off
  Reset : Outport
  wires:
  Delay/1 -> Delay One Step/2
  Constant6/1 -> GreaterThanOrEqual/1
  Delay One Step/1 -> Add1/2, GreaterThanOrEqual/2
  GreaterThanOrEqual/1 -> Reset/1, Delay/1, Switch1/2
  Constant1/1 -> Switch1/1
  Add1/1 -> Delay One Step/1
  Constant2/1 -> Switch1/3
  Switch1/1 -> Add1/1

== system Final_Tune_of_Bandwidth_PI_Result/Subsystem3/PLL2/PhaseMaximumDetector2/CycleDetector ==
  Enable : EnablePort
  Add1 : Sum
  Constant1 : Constant  Value=single(0)
  Constant2 : Constant  Value=single(1)
  Constant6 : Constant  Value=single(2)
  Delay : Delay  DelayLength=1
  Delay One Step : Delay  DelayLength=1  ExternalReset=Rising
      settings: InputPortMap=u0,r5
  GreaterThanOrEqual : RelationalOperator  Operator===  OutDataTypeStr=boolean  RndMeth=Simplest  InputSameDT=off
  Switch1 : Switch  Criteria=u2 > Threshold  SaturateOnIntegerOverflow=off  InputSameDT=off
  Reset : Outport
  wires:
  Delay/1 -> Delay One Step/2
  Constant6/1 -> GreaterThanOrEqual/1
  Delay One Step/1 -> Add1/2, GreaterThanOrEqual/2
  GreaterThanOrEqual/1 -> Reset/1, Delay/1, Switch1/2
  Constant1/1 -> Switch1/1
  Add1/1 -> Delay One Step/1
  Constant2/1 -> Switch1/3
  Switch1/1 -> Add1/1

== system Final_Tune_of_Bandwidth_PI_Result/Subsystem3/PLL_Loop1/SOGI 1st/Integrator ==
  In : Inport
  Delay1 : Delay  DelayLength=1
  Delay2 : Delay  DelayLength=1
  Delay3 : Delay  DelayLength=1
  Gain : Gain  Gain=100e-6/12
  Gain1 : Gain  Gain=23
  Gain2 : Gain  Gain=16
  Gain3 : Gain  Gain=5
  Sum : Sum  Inputs=|+-
  Sum1 : Sum  Inputs=|++
  Sum2 : Sum  Inputs=|++
  Out : Outport
  wires:
  Delay2/1 -> Gain2/1, Delay3/1
  Delay1/1 -> Sum2/2, Gain1/1, Delay2/1
  Delay3/1 -> Gain3/1
  Gain2/1 -> Sum/2
  Gain1/1 -> Sum/1
  Gain3/1 -> Sum1/2
  Sum/1 -> Sum1/1
  Gain/1 -> Sum2/1
  Sum2/1 -> Delay1/1
  In/1 -> Gain/1
  Sum1/1 -> Out/1

== system Final_Tune_of_Bandwidth_PI_Result/Subsystem3/PLL_Loop1/SOGI 1st/Integrator1 ==
  In : Inport
  Delay1 : Delay  DelayLength=1
  Delay2 : Delay  DelayLength=1
  Delay3 : Delay  DelayLength=1
  Gain : Gain  Gain=100e-6/12
  Gain1 : Gain  Gain=23
  Gain2 : Gain  Gain=16
  Gain3 : Gain  Gain=5
  Sum : Sum  Inputs=|+-
  Sum1 : Sum  Inputs=|++
  Sum2 : Sum  Inputs=|++
  Out : Outport
  wires:
  Delay2/1 -> Gain2/1, Delay3/1
  Delay1/1 -> Sum2/2, Gain1/1, Delay2/1
  Delay3/1 -> Gain3/1
  Gain2/1 -> Sum/2
  Gain1/1 -> Sum/1
  Gain3/1 -> Sum1/2
  Sum/1 -> Sum1/1
  Gain/1 -> Sum2/1
  Sum2/1 -> Delay1/1
  In/1 -> Gain/1
  Sum1/1 -> Out/1

== system Final_Tune_of_Bandwidth_PI_Result/Subsystem3/PLL_Loop1/SOGI 1st/Integrator2 ==
  In : Inport
  Delay1 : Delay  DelayLength=1
  Delay2 : Delay  DelayLength=1
  Delay3 : Delay  DelayLength=1
  Gain : Gain  Gain=100e-6/12
  Gain1 : Gain  Gain=23
  Gain2 : Gain  Gain=16
  Gain3 : Gain  Gain=5
  Sum : Sum  Inputs=|+-
  Sum1 : Sum  Inputs=|++
  Sum2 : Sum  Inputs=|++
  Out : Outport
  wires:
  In/1 -> Gain/1
  Delay2/1 -> Gain2/1, Delay3/1
  Delay1/1 -> Sum2/2, Gain1/1, Delay2/1
  Delay3/1 -> Gain3/1
  Gain2/1 -> Sum/2
  Gain1/1 -> Sum/1
  Gain3/1 -> Sum1/2
  Sum/1 -> Sum1/1
  Sum1/1 -> Out/1
  Gain/1 -> Sum2/1
  Sum2/1 -> Delay1/1

== system Final_Tune_of_Bandwidth_PI_Result/Subsystem3/PLL_Loop1/SOGI 1st3/Integrator ==
  In : Inport
  Delay1 : Delay  DelayLength=1
  Delay2 : Delay  DelayLength=1
  Delay3 : Delay  DelayLength=1
  Gain : Gain  Gain=100e-6/12
  Gain1 : Gain  Gain=23
  Gain2 : Gain  Gain=16
  Gain3 : Gain  Gain=5
  Sum : Sum  Inputs=|+-
  Sum1 : Sum  Inputs=|++
  Sum2 : Sum  Inputs=|++
  Out : Outport
  wires:
  Delay2/1 -> Gain2/1, Delay3/1
  Delay1/1 -> Sum2/2, Gain1/1, Delay2/1
  Delay3/1 -> Gain3/1
  Gain2/1 -> Sum/2
  Gain1/1 -> Sum/1
  Gain3/1 -> Sum1/2
  Sum/1 -> Sum1/1
  Gain/1 -> Sum2/1
  Sum2/1 -> Delay1/1
  In/1 -> Gain/1
  Sum1/1 -> Out/1

== system Final_Tune_of_Bandwidth_PI_Result/Subsystem3/PLL_Loop1/SOGI 1st3/Integrator1 ==
  In : Inport
  Delay1 : Delay  DelayLength=1
  Delay2 : Delay  DelayLength=1
  Delay3 : Delay  DelayLength=1
  Gain : Gain  Gain=100e-6/12
  Gain1 : Gain  Gain=23
  Gain2 : Gain  Gain=16
  Gain3 : Gain  Gain=5
  Sum : Sum  Inputs=|+-
  Sum1 : Sum  Inputs=|++
  Sum2 : Sum  Inputs=|++
  Out : Outport
  wires:
  Delay2/1 -> Gain2/1, Delay3/1
  Delay1/1 -> Sum2/2, Gain1/1, Delay2/1
  Delay3/1 -> Gain3/1
  Gain2/1 -> Sum/2
  Gain1/1 -> Sum/1
  Gain3/1 -> Sum1/2
  Sum/1 -> Sum1/1
  Gain/1 -> Sum2/1
  Sum2/1 -> Delay1/1
  In/1 -> Gain/1
  Sum1/1 -> Out/1

== system Final_Tune_of_Bandwidth_PI_Result/Subsystem3/PLL_Loop1/SOGI 1st3/Integrator2 ==
  In : Inport
  Delay1 : Delay  DelayLength=1
  Delay2 : Delay  DelayLength=1
  Delay3 : Delay  DelayLength=1
  Gain : Gain  Gain=100e-6/12
  Gain1 : Gain  Gain=23
  Gain2 : Gain  Gain=16
  Gain3 : Gain  Gain=5
  Sum : Sum  Inputs=|+-
  Sum1 : Sum  Inputs=|++
  Sum2 : Sum  Inputs=|++
  Out : Outport
  wires:
  In/1 -> Gain/1
  Delay2/1 -> Gain2/1, Delay3/1
  Delay1/1 -> Sum2/2, Gain1/1, Delay2/1
  Delay3/1 -> Gain3/1
  Gain2/1 -> Sum/2
  Gain1/1 -> Sum/1
  Gain3/1 -> Sum1/2
  Sum/1 -> Sum1/1
  Sum1/1 -> Out/1
  Gain/1 -> Sum2/1
  Sum2/1 -> Delay1/1

== stateflow chart Final_Tune_of_Bandwidth_PI_Result/Subsystem3/PLL_Loop/Chart ==
  (default) -> (junction 2)
  (junction 2) -> (junction 40)
  (junction 40) -> (junction 41) [order 1] : [Angle_State>= 2*pi]
  (junction 40) -> (junction 42) [order 2]
  (junction 41) -> (junction 46) : {
      | resetVal = Angle_State - 2*pi;
      | trigVal = 1;
      | }
  (junction 42) -> (junction 43) [order 1] : [Angle_State < 0]
  (junction 42) -> (junction 44) [order 2] : {resetVal = 0;
      | trigVal = 0;}
  (junction 43) -> (junction 45) : {
      | resetVal = Angle_State + 2*pi;
      | trigVal = 1;
      | }
  (junction 45) -> (junction 44)
  (junction 46) -> (junction 45)
  (junction 44) -> (junction 14)
  data: Angle_State input single; trigVal output single; resetVal output single

== stateflow chart Final_Tune_of_Bandwidth_PI_Result/Chart1 ==
  state GPin_FC [parallel]
    settings: executionOrder=1
    state Rate_100us
      on every(1,tic): send(GPin_FC);
    (default) -> GPin_FC.Rate_100us : /{send(GPin_FC);}
  state ADC_FC [parallel]
    settings: executionOrder=2
    state Rate_100us
      on every(1,tic): send(ADC_FC);
    (default) -> ADC_FC.Rate_100us : /{send(ADC_FC);}
  state PLL_FC [parallel]
    settings: executionOrder=3
    state Rate_100us
      on every(1,tic): send(PLL_FC);
    (default) -> PLL_FC.Rate_100us : /{send(PLL_FC);}
  state CurrentLoop_FC [parallel]
    settings: executionOrder=4
    state Rate_100us
      on every(1,tic): send(CurrentLoop_FC);
    (default) -> CurrentLoop_FC.Rate_100us : /{send(CurrentLoop_FC);}
  state VoltageLoop_FC [parallel]
    settings: executionOrder=5
    state Rate_1000us
      on every(10,tic): send(VoltageLoop_FC);
    (default) -> Rate_1000us : /{send(VoltageLoop_FC);}
  state GPout_FC [parallel]
    settings: executionOrder=6
    state Rate_100us
      on every(1,tic): send(GPout_FC);
    (default) -> GPout_FC.Rate_100us : /{send(GPout_FC);}
  events: ADC_FC output FUNCTION_CALL_EVENT; PLL_FC output FUNCTION_CALL_EVENT; tic input FUNCTION_CALL_EVENT; CurrentLoop_FC output FUNCTION_CALL_EVENT; VoltageLoop_FC output FUNCTION_CALL_EVENT; GPin_FC output FUNCTION_CALL_EVENT; GPout_FC output FUNCTION_CALL_EVENT
